simulink model "CAMFC2_04_simple_DoubleIntegrator_02"  (R2017b)
settings: Solver=ode23  StartTime=0.0  StopTime=200  RelTol=1e-3  EnableMultiTasking=on
InitFcn:
  | constant_CAMFC2_04_Simple_DoubleIntegrator_02
values from neighbouring files (symbols this model uses):
  alpha = 0.1    [constant_CAMFC2_01_WMR01.m]    (also in constant_CAMFC2_04_Comp.m = 0.01; constant_CAMFC2_04_Quad_03.m; constant_CAMFC2_04_Simple.m = 0.01; constant_CAMFC2_04_Simple_DoubleIntegrator.m = 0.01)
  AN = [     0 1 0 0 ... (first row only)    [constant_CAMFC2_01_WMR01.m]    (also in constant_CAMFC2_04_Comp.m = [     0 1 0 0 1; constant_CAMFC2_04_Quad_03.m; constant_CAMFC2_04_Simple.m; constant_CAMFC2_04_Simple_DoubleIntegrator.m)
  BN = [     1 0 0 0 ... (first row only)    [constant_CAMFC2_01_WMR01.m]    (also in constant_CAMFC2_04_Comp.m = [     0 0 0 0 0; constant_CAMFC2_04_Quad_03.m; constant_CAMFC2_04_Simple.m; constant_CAMFC2_04_Simple_DoubleIntegrator.m)
  Bp = 0.01    [constant_CAMFC2_04_Comp.m]    (also in constant_CAMFC2_04_Simple.m; constant_CAMFC2_04_Simple_DoubleIntegrator.m; constant_CAMFC2_04_Simple_DoubleIntegrator_02.m; constants_CAMFC2_Pendulum_Comp_Lewis.m)
  chi = [0 0 0 0 ... (first row only)    [constant_CAMFC2_01_WMR01.m]    (also in constant_CAMFC2_04_Comp.m = X_m*ones(n0,1); constant_CAMFC2_04_Quad_03.m = X_m*ones(n0,1); constant_CAMFC2_04_Simple.m = X_m*ones(n0,1); constant_CAMFC2_04_Simple_DoubleIntegrator.m = X_m*ones(n0,1))
  Disturb_Freq = 2    [constant_CAMFC2_04_Comp.m]    (also in constant_CAMFC2_04_Simple.m; constant_CAMFC2_04_Simple_DoubleIntegrator.m; constant_CAMFC2_04_Simple_DoubleIntegrator_02.m; constants_CAMFC2_Pendulum_Comp_Lewis.m)
  Disturb_Val = 1    [constant_CAMFC2_04_Comp.m]    (also in constant_CAMFC2_04_Simple.m; constant_CAMFC2_04_Simple_DoubleIntegrator.m; constant_CAMFC2_04_Simple_DoubleIntegrator_02.m; constants_CAMFC2_Pendulum_Comp_Lewis.m)
  epsilon_struct = struct('data',epsilon_InitVal)    [constant_CAMFC2_01_WMR01.m]    (also in constant_CAMFC2_04_Comp.m; constant_CAMFC2_04_Quad_03.m; constant_CAMFC2_04_Simple.m; constant_CAMFC2_04_Simple_DoubleIntegrator.m)
  gama1_Int1 = 1e+2*1e0    (= 100)    [constant_CAMFC2_04_Simple_DoubleIntegrator.m]    (also in constant_CAMFC2_04_Simple_DoubleIntegrator_02.m)
  gama1_Int2 = 1e+3*1e0    (= 1000)    [constant_CAMFC2_04_Simple_DoubleIntegrator.m]    (also in constant_CAMFC2_04_Simple_DoubleIntegrator_02.m)
  gama2_Int1 = 1e+0*1e0    (= 1)    [constant_CAMFC2_04_Simple_DoubleIntegrator.m]    (also in constant_CAMFC2_04_Simple_DoubleIntegrator_02.m)
  gama2_Int2 = 1e+2*1e0    (= 100)    [constant_CAMFC2_04_Simple_DoubleIntegrator.m]    (also in constant_CAMFC2_04_Simple_DoubleIntegrator_02.m)
  ge = 9.81    [constant_CAMFC2_04_Comp.m]    (also in constant_CAMFC2_04_Quad_03.m; constant_CAMFC2_04_Simple.m; constant_CAMFC2_04_Simple_DoubleIntegrator.m; constant_CAMFC2_04_Simple_DoubleIntegrator_02.m)
  H = L + BN    [constant_CAMFC2_01_WMR01.m]    (also in constant_CAMFC2_04_Comp.m; constant_CAMFC2_04_Quad_03.m; constant_CAMFC2_04_Simple.m; constant_CAMFC2_04_Simple_DoubleIntegrator.m)
  Jp = 1    [constant_CAMFC2_04_Comp.m]    (also in constant_CAMFC2_04_Simple.m; constant_CAMFC2_04_Simple_DoubleIntegrator.m; constant_CAMFC2_04_Simple_DoubleIntegrator_02.m; constants_CAMFC2_Pendulum_Comp_Lewis.m)
  k1 = 1    [constant_CAMFC2_01_WMR01.m]    (also in constant_CAMFC2_04_Comp.m; constant_CAMFC2_04_Quad_03.m = 50; constant_CAMFC2_04_Simple.m; constant_CAMFC2_04_Simple_DoubleIntegrator.m)
  k2 = 1    [constant_CAMFC2_01_WMR01.m]    (also in constant_CAMFC2_04_Comp.m; constant_CAMFC2_04_Quad_03.m; constant_CAMFC2_04_Simple.m; constant_CAMFC2_04_Simple_DoubleIntegrator.m)
  lp = 0.1    [constant_CAMFC2_04_Comp.m]    (also in constant_CAMFC2_04_Simple.m; constant_CAMFC2_04_Simple_DoubleIntegrator.m; constant_CAMFC2_04_Simple_DoubleIntegrator_02.m; constants_CAMFC2_Pendulum_Comp_Lewis.m)
  Mp = 0.1    [constant_CAMFC2_04_Comp.m]    (also in constant_CAMFC2_04_Simple.m; constant_CAMFC2_04_Simple_DoubleIntegrator.m; constant_CAMFC2_04_Simple_DoubleIntegrator_02.m; constants_CAMFC2_Pendulum_Comp_Lewis.m)
  n = 4    [constant_CAMFC2_01_WMR01.m]    (also in constant_CAMFC2_04_Comp.m = 2; constant_CAMFC2_04_Quad_03.m = 6; constant_CAMFC2_04_Simple.m = 2; constant_CAMFC2_04_Simple_DoubleIntegrator.m = 2)
  N = 4    [constant_CAMFC2_01_WMR01.m]    (also in constant_CAMFC2_04_Comp.m = 5; constant_CAMFC2_04_Quad_03.m; constant_CAMFC2_04_Simple.m; constant_CAMFC2_04_Simple_DoubleIntegrator.m)
  n0 = 2    [constant_CAMFC2_01_WMR01.m]    (also in constant_CAMFC2_04_Comp.m = 1; constant_CAMFC2_04_Quad_03.m = 3; constant_CAMFC2_04_Simple.m; constant_CAMFC2_04_Simple_DoubleIntegrator.m = 1)
  Observer_Gain = 100    [constant_CAMFC2_01_WMR01.m]    (also in constant_CAMFC2_04_Comp.m = 10; constant_CAMFC2_04_Quad_03.m = 1; constant_CAMFC2_04_Simple.m; constant_CAMFC2_04_Simple_DoubleIntegrator.m)
  Observer_Gain1 = 100    [constant_CAMFC2_01_WMR01.m]    (also in constant_CAMFC2_04_Comp.m = 10; constant_CAMFC2_04_Quad_03.m = 1; constant_CAMFC2_04_Simple.m; constant_CAMFC2_04_Simple_DoubleIntegrator.m)
  Omega = [0 0 ... (first row only)    [constant_CAMFC2_04_Comp.m]    (also in constant_CAMFC2_04_Simple.m; constant_CAMFC2_04_Simple_DoubleIntegrator.m; constant_CAMFC2_04_Simple_DoubleIntegrator_02.m; constant_CAMFC2_04_Simple_Formation.m)
  P_struct = struct('data',P_InitVal)    [constant_CAMFC2_01_WMR01.m]    (also in constant_CAMFC2_04_Comp.m; constant_CAMFC2_04_Quad_03.m; constant_CAMFC2_04_Simple.m; constant_CAMFC2_04_Simple_DoubleIntegrator.m)
  Q_Int2 = 1.0e+1    (= 10)    [constant_CAMFC2_04_Simple_DoubleIntegrator.m]    (also in constant_CAMFC2_04_Simple_DoubleIntegrator_02.m = 2)
  rho1 = 1e-1    (= 0.1)    [constant_CAMFC2_01_WMR01.m]    (also in constant_CAMFC2_04_Comp.m = 1; constant_CAMFC2_04_Quad_03.m = 1; constant_CAMFC2_04_Simple.m = 1; constant_CAMFC2_04_Simple_DoubleIntegrator.m = 1)
  rho2 = 1e-3    (= 0.001)    [constant_CAMFC2_01_WMR01.m]    (also in constant_CAMFC2_04_Comp.m = 1; constant_CAMFC2_04_Quad_03.m = 1; constant_CAMFC2_04_Simple.m = 1; constant_CAMFC2_04_Simple_DoubleIntegrator.m = 10)
  T_struct = struct('data',T_InitVal)    [constant_CAMFC2_01_WMR01.m]    (also in constant_CAMFC2_04_Comp.m; constant_CAMFC2_04_Quad_03.m; constant_CAMFC2_04_Simple.m; constant_CAMFC2_04_Simple_DoubleIntegrator.m)
  Upsilon_M = Upsilon_m*ones(n,1)    [constant_CAMFC2_01_WMR01.m]    (also in constant_CAMFC2_04_Comp.m; constant_CAMFC2_04_Quad_03.m = Upsilon_m*ones(n0,1); constant_CAMFC2_04_Simple.m; constant_CAMFC2_04_Simple_DoubleIntegrator.m)
(part 1 of 4)
settings Model: ExtModeTrigDuration=100  Creator=hp  LastModifiedBy=ali.safaei
settings DataIOCC: LimitDataPoints=on  SaveFinalState=on  SaveFormat=StructureWithTime  SaveOutput=off  SaveState=on  StateSaveName=tmp_raccel_xout  SignalLoggingName=tmp_raccel_logsout
settings OptimizationCC: EfficientMapNaN2IntZero=off  LifeSpan=inf
settings DebuggingCC: UnderspecifiedInitializationDetection=Classic  MergeDetectMultiDrivingBlocksExec=none  SFUnexpectedBacktrackingDiag=warning  SFNoUnconditionalDefaultTransitionDiag=warning  SFExecutionAtInitializationDiag=none
settings HardwareCC: ProdBitPerPointer=32  ProdBitPerSizeT=32  ProdBitPerPtrDiffT=32  ProdLargestAtomicFloat=None  ProdIntDivRoundTo=Undefined  ProdEndianess=Unspecified  ProdWordSize=32  ProdHWDeviceType=32-bit Generic  TargetBitPerPointer=64  TargetBitPerSizeT=64  TargetBitPerPtrDiffT=64  TargetLongLongMode=on  TargetIntDivRoundTo=Zero  TargetEndianess=LittleEndian  TargetWordSize=64  TargetHWDeviceType=MATLAB Host  ProdEqTarget=off
settings ModelReferenceCC: PropagateSignalLabelsOutOfModel=off
settings RTWCC: SystemTargetFile=raccel.tlc  TemplateMakefile=raccel_default_tmf  RTWVerbose=off  RTWUseSimCustomCode=on
settings CodeAppCC: GenerateComments=off  MaxIdLength=128  MangleLength=10  SimulinkBlockComments=off
settings RaccelTargetCC: GeneratePreprocessorConditionals=Use local settings  MultiInstanceERTCode=off  ExtModeMexArgs='', 0, 54523  ENABLE_SLEXEC_SSBRIDGE=0  RTWCAPIParams=on
settings ConfigComp: CovMetricSettings=dw  CovHtmlReporting=on  CovSaveCumulativeToWorkspaceVar=on  CovSaveSingleToWorkspaceVar=on  CovExternalEMLEnable=off

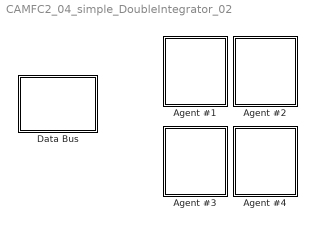
== system CAMFC2_04_simple_DoubleIntegrator_02 ==
  Agent #1 : Subsystem
  Agent #2 : Subsystem
  Agent #3 : Subsystem
  Agent #4 : Subsystem
  "Data Bus " : Subsystem

== system CAMFC2_04_simple_DoubleIntegrator_02/Agent #1 ==
  Agent # : Constant
  Controller interpreter #1 : MATLAB Function  TreatAsAtomicUnit=on
  Decenteralized Cooperaive Controller #1 : Subsystem
  Pendulum Plant #1 : Subsystem
  tag scope: u1=global, x1=global
  wires:
  Decenteralized Cooperaive Controller #1/1(U1) -> Controller interpreter #1/1(U)
  Agent #/1 -> Decenteralized Cooperaive Controller #1/1(Agent_Num)
  Pendulum Plant #1/1(Y) -> [x1]
  Controller interpreter #1/1(u) -> [u1], Pendulum Plant #1/1(U)

== system CAMFC2_04_simple_DoubleIntegrator_02/Agent #2 ==
  Agent # : Constant  Value=2
  Controller interpreter #2 : MATLAB Function  TreatAsAtomicUnit=on
  Decenteralized Cooperaive Controller #2 : Subsystem
  Pendulum Plant #2 : Subsystem
  tag scope: u2=global, x2=global
  wires:
  Controller interpreter #2/1(u) -> Pendulum Plant #2/1(U), [u2]
  Pendulum Plant #2/1(Y) -> [x2]
  Agent #/1 -> Decenteralized Cooperaive Controller #2/1(Agent_Num)
  Decenteralized Cooperaive Controller #2/1(U2) -> Controller interpreter #2/1(U)

== system CAMFC2_04_simple_DoubleIntegrator_02/Agent #3 ==
  Agent # : Constant  Value=3
  Controller interpreter #3 : MATLAB Function  TreatAsAtomicUnit=on
  Decenteralized Cooperaive Controller #3 : Subsystem
  Pendulum Plant #3 : Subsystem
  tag scope: u3=global, x3=global
  wires:
  Decenteralized Cooperaive Controller #3/1(U3) -> Controller interpreter #3/1(U)
  Agent #/1 -> Decenteralized Cooperaive Controller #3/1(Agent_Num)
  Pendulum Plant #3/1(Y) -> [x3]
  Controller interpreter #3/1(u) -> [u3], Pendulum Plant #3/1(U)

== system CAMFC2_04_simple_DoubleIntegrator_02/Agent #4 ==
  Agent # : Constant  Value=4
  Controller interpreter #4 : MATLAB Function  TreatAsAtomicUnit=on
  Decenteralized Cooperaive Controller #4 : Subsystem
  Pendulum Plant #4 : Subsystem
  tag scope: u4=global, x4=global
  wires:
  Controller interpreter #4/1(u) -> Pendulum Plant #4/1(U), [u4]
  Pendulum Plant #4/1(Y) -> [x4]
  Agent #/1 -> Decenteralized Cooperaive Controller #4/1(Agent_Num)
  Decenteralized Cooperaive Controller #4/1(U4) -> Controller interpreter #4/1(U)

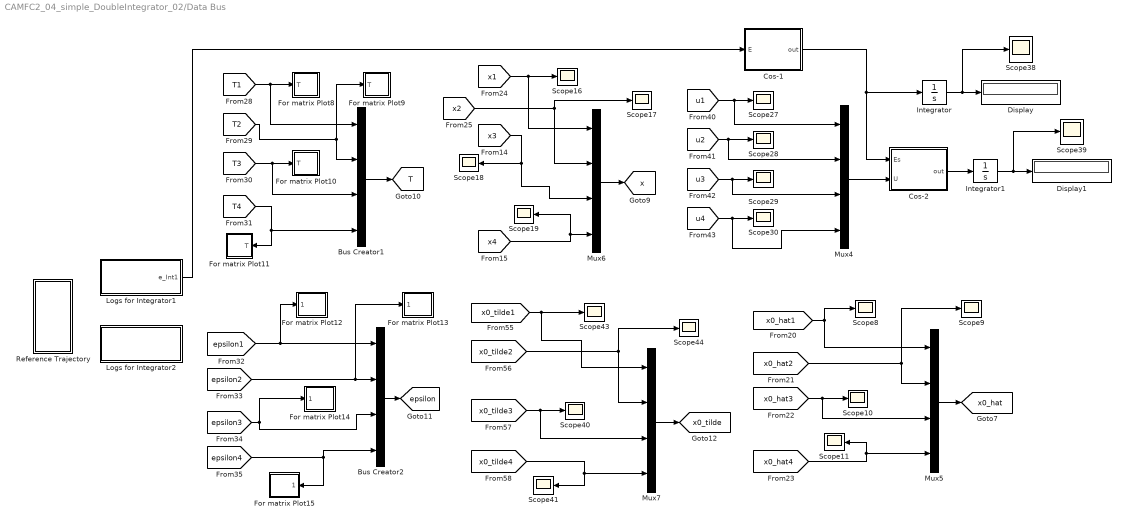
== system CAMFC2_04_simple_DoubleIntegrator_02/Data Bus  ==
  Bus Creator1 : BusCreator  Inputs=4  OutDataTypeStr=Bus: T_bus
  Bus Creator2 : BusCreator  Inputs=4  OutDataTypeStr=Bus: epsilon_bus
  Cos-1 : MATLAB Function  TreatAsAtomicUnit=on
  Cos-2 : MATLAB Function  TreatAsAtomicUnit=on
  Display : Display
  Display1 : Display
  For matrix Plot10 : Subsystem
  For matrix Plot11 : Subsystem
  For matrix Plot12 : Subsystem
  For matrix Plot13 : Subsystem
  For matrix Plot14 : Subsystem
  For matrix Plot15 : Subsystem
  For matrix Plot8 : Subsystem
  For matrix Plot9 : Subsystem
  Integrator : Integrator
  Integrator1 : Integrator
  Logs for Integrator1 : Subsystem
  Logs for Integrator2 : Subsystem
  Mux{4..7} (4 alike) : Mux
  Reference Trajectory : Subsystem
  Scope{8..11,16..19,27..30,38..41,43..44} (18 alike) : Scope
  tag scope: T=global, epsilon=global, x0_hat=global, x0_tilde=global, x=global
  wires:
  [x0_hat2] -> Scope9/1, Mux5/2
  [x0_hat1] -> Scope8/1, Mux5/1
  Mux5/1 -> [x0_hat]
  [x2] -> Scope17/1, Mux6/2
  [x1] -> Mux6/1, Scope16/1
  Mux6/1 -> [x]
  [x3] -> Scope18/1, Mux6/3
  [x4] -> Scope19/1, Mux6/4
  [x0_hat3] -> Mux5/3, Scope10/1
  [x0_hat4] -> Mux5/4, Scope11/1
  [T2] -> For matrix Plot9/1(T), Bus Creator1/2
  [T1] -> Bus Creator1/1, For matrix Plot8/1(T)
  Bus Creator1/1 -> [T]
  [T3] -> Bus Creator1/3, For matrix Plot10/1(T)
  [T4] -> Bus Creator1/4, For matrix Plot11/1(T)
  [epsilon2] -> For matrix Plot13/1(epsilon), Bus Creator2/2
  [epsilon1] -> For matrix Plot12/1(epsilon), Bus Creator2/1
  Bus Creator2/1 -> [epsilon]
  [epsilon3] -> For matrix Plot14/1(epsilon), Bus Creator2/3
  [epsilon4] -> Bus Creator2/4, For matrix Plot15/1(epsilon)
  [u2] -> Mux4/2, Scope28/1
  [u1] -> Mux4/1, Scope27/1
  [u4] -> Mux4/4, Scope30/1
  [u3] -> Mux4/3, Scope29/1
  [x0_tilde4] -> Mux7/4, Scope41/1
  [x0_tilde1] -> Mux7/1, Scope43/1
  [x0_tilde3] -> Mux7/3, Scope40/1
  [x0_tilde2] -> Mux7/2, Scope44/1
  Mux7/1 -> [x0_tilde]
  Cos-2/1(out) -> Integrator1/1
  Integrator1/1 -> Display1/1, Scope39/1
  Logs for Integrator1/1(e_Int1) -> Cos-1/1(E)
  Cos-1/1(out) -> Cos-2/1(Es), Integrator/1
  Mux4/1 -> Cos-2/2(U)
  Integrator/1 -> Scope38/1, Display/1

== system CAMFC2_04_simple_DoubleIntegrator_02/Agent #1/Decenteralized Cooperaive Controller #1 ==
  Agent_Num : Inport
  Cooperative observer for formation variables #1 : Subsystem
  Cooperative observer for leader states #1 : Subsystem
  Differentiator1 : Subsystem
  First Integrator #1 : Subsystem
  Second Integrator #1 : Subsystem
  formation topology for second integrator : MATLAB Function  TreatAsAtomicUnit=on
  U1 : Outport
  tag scope: U1_Int1=global
  wires:
  Agent_Num/1 -> Cooperative observer for leader states #1/1(Agent_Num), Cooperative observer for formation variables #1/1(Agent_Num), First Integrator #1/1(Agent Num), Second Integrator #1/1(Agent_Num)
  Second Integrator #1/1(U) -> U1/1
  Cooperative observer for leader states #1/1(x0_hat_i) -> Differentiator1/1(x_d), First Integrator #1/2(x0_hat_i)
  Cooperative observer for formation variables #1/1(T_i) -> formation topology for second integrator/1(T_i), First Integrator #1/3(T_i)
  First Integrator #1/1(U to Second Integrator) -> [U1_Int1]
  [U_Int1] -> formation topology for second integrator/2(U_Int1)
  formation topology for second integrator/1(New_T_i) -> Second Integrator #1/3(T_i)
  Differentiator1/1(Dx_d) -> Second Integrator #1/2(Dx0_hat_i)

== system CAMFC2_04_simple_DoubleIntegrator_02/Agent #1/Pendulum Plant #1 ==
  U : Inport
  Plant : Subsystem
  Y : Outport
  wires:
  U/1 -> Plant/1(U)
  Plant/1(Y) -> Y/1

== system CAMFC2_04_simple_DoubleIntegrator_02/Agent #2/Decenteralized Cooperaive Controller #2 ==
  Agent_Num : Inport
  Cooperative observer for formation variables #2 : Subsystem
  Cooperative observer for leader states #2 : Subsystem
  Differentiator1 : Subsystem
  First Integrator #2 : Subsystem
  Second Integrator #2 : Subsystem
  formation topology for second integrator : MATLAB Function  TreatAsAtomicUnit=on
  U2 : Outport
  tag scope: U2_Int1=global
  wires:
  Cooperative observer for leader states #2/1(x0_hat_i) -> Differentiator1/1(x_d), First Integrator #2/2(x0_hat_i)
  Second Integrator #2/1(U) -> U2/1
  Agent_Num/1 -> Cooperative observer for formation variables #2/1(Agent_Num), Cooperative observer for leader states #2/1(Agent_Num), First Integrator #2/1(Agent Num), Second Integrator #2/1(Agent_Num)
  First Integrator #2/1(U to Second Integrator) -> [U2_Int1]
  formation topology for second integrator/1(New_T_i) -> Second Integrator #2/3(T_i)
  Cooperative observer for formation variables #2/1(T_i) -> First Integrator #2/3(T_i), formation topology for second integrator/1(T_i)
  [U_Int1] -> formation topology for second integrator/2(U_Int1)
  Differentiator1/1(Dx_d) -> Second Integrator #2/2(Dx0_hat_i)

== system CAMFC2_04_simple_DoubleIntegrator_02/Agent #2/Pendulum Plant #2 ==
  U : Inport
  Plant : Subsystem
  Y : Outport
  wires:
  Plant/1(Y) -> Y/1
  U/1 -> Plant/1(U)

== system CAMFC2_04_simple_DoubleIntegrator_02/Agent #3/Decenteralized Cooperaive Controller #3 ==
  Agent_Num : Inport
  Cooperative observer for formation variables #3 : Subsystem
  Cooperative observer for leader states #3 : Subsystem
  Differentiator1 : Subsystem
  First Integrator #3 : Subsystem
  Second Integrator #3 : Subsystem
  formation topology for second integrator : MATLAB Function  TreatAsAtomicUnit=on
  U3 : Outport
  tag scope: U3_Int1=global
  wires:
  Agent_Num/1 -> Cooperative observer for leader states #3/1(Agent_Num), Cooperative observer for formation variables #3/1(Agent_Num), First Integrator #3/1(Agent Num), Second Integrator #3/1(Agent_Num)
  Second Integrator #3/1(U) -> U3/1
  Cooperative observer for leader states #3/1(x0_hat_i) -> Differentiator1/1(x_d), First Integrator #3/2(x0_hat_i)
  First Integrator #3/1(U to Second Integrator) -> [U3_Int1]
  formation topology for second integrator/1(New_T_i) -> Second Integrator #3/3(T_i)
  Cooperative observer for formation variables #3/1(T_i) -> First Integrator #3/3(T_i), formation topology for second integrator/1(T_i)
  [U_Int1] -> formation topology for second integrator/2(U_Int1)
  Differentiator1/1(Dx_d) -> Second Integrator #3/2(Dx0_hat_i)

== system CAMFC2_04_simple_DoubleIntegrator_02/Agent #3/Pendulum Plant #3 ==
  U : Inport
  Plant : Subsystem
  Y : Outport
  wires:
  U/1 -> Plant/1(U)
  Plant/1(Y) -> Y/1

== system CAMFC2_04_simple_DoubleIntegrator_02/Agent #4/Decenteralized Cooperaive Controller #4 ==
  Agent_Num : Inport
  Cooperative observer for formation variables #4 : Subsystem
  Cooperative observer for leader states #4 : Subsystem
  Differentiator1 : Subsystem
  First Integrator #4 : Subsystem
  Second Integrator #4 : Subsystem
  formation topology for second integrator : MATLAB Function  TreatAsAtomicUnit=on
  U4 : Outport
  tag scope: U4_Int1=global
  wires:
  Cooperative observer for leader states #4/1(x0_hat_i) -> Differentiator1/1(x_d), First Integrator #4/2(x0_hat_i)
  Second Integrator #4/1(U) -> U4/1
  Agent_Num/1 -> First Integrator #4/1(Agent Num), Cooperative observer for formation variables #4/1(Agent_Num), Cooperative observer for leader states #4/1(Agent_Num), Second Integrator #4/1(Agent_Num)
  First Integrator #4/1(U to Second Integrator) -> [U4_Int1]
  formation topology for second integrator/1(New_T_i) -> Second Integrator #4/3(T_i)
  Cooperative observer for formation variables #4/1(T_i) -> First Integrator #4/3(T_i), formation topology for second integrator/1(T_i)
  [U_Int1] -> formation topology for second integrator/2(U_Int1)
  Differentiator1/1(Dx_d) -> Second Integrator #4/2(Dx0_hat_i)

== system CAMFC2_04_simple_DoubleIntegrator_02/Agent #4/Pendulum Plant #4 ==
  U : Inport
  Plant : Subsystem
  Y : Outport
  wires:
  Plant/1(Y) -> Y/1
  U/1 -> Plant/1(U)

== system CAMFC2_04_simple_DoubleIntegrator_02/Data Bus /For matrix Plot10 ==
  T : Inport
  MATLAB Function : MATLAB Function  TreatAsAtomicUnit=on
  To Workspace : ToWorkspace  VariableName=T3  SaveFormat=Structure With Time  SampleTime=-1
  wires:
  T/1 -> MATLAB Function/1(u)
  MATLAB Function/1(y) -> To Workspace/1

== system CAMFC2_04_simple_DoubleIntegrator_02/Data Bus /For matrix Plot11 ==
  T : Inport
  MATLAB Function : MATLAB Function  TreatAsAtomicUnit=on
  To Workspace : ToWorkspace  VariableName=T4  SaveFormat=Structure With Time  SampleTime=-1
  wires:
  MATLAB Function/1(y) -> To Workspace/1
  T/1 -> MATLAB Function/1(u)

== system CAMFC2_04_simple_DoubleIntegrator_02/Data Bus /For matrix Plot12 ==
  epsilon : Inport
  MATLAB Function : MATLAB Function  TreatAsAtomicUnit=on
  To Workspace : ToWorkspace  VariableName=epsilon1  SaveFormat=Structure With Time  SampleTime=-1
  wires:
  epsilon/1 -> MATLAB Function/1(u)
  MATLAB Function/1(y) -> To Workspace/1

== system CAMFC2_04_simple_DoubleIntegrator_02/Data Bus /For matrix Plot13 ==
  epsilon : Inport
  MATLAB Function : MATLAB Function  TreatAsAtomicUnit=on
  To Workspace : ToWorkspace  VariableName=epsilon2  SaveFormat=Structure With Time  SampleTime=-1
  wires:
  MATLAB Function/1(y) -> To Workspace/1
  epsilon/1 -> MATLAB Function/1(u)

== system CAMFC2_04_simple_DoubleIntegrator_02/Data Bus /For matrix Plot14 ==
  epsilon : Inport
  MATLAB Function : MATLAB Function  TreatAsAtomicUnit=on
  To Workspace : ToWorkspace  VariableName=epsilon3  SaveFormat=Structure With Time  SampleTime=-1
  wires:
  MATLAB Function/1(y) -> To Workspace/1
  epsilon/1 -> MATLAB Function/1(u)

== system CAMFC2_04_simple_DoubleIntegrator_02/Data Bus /For matrix Plot15 ==
  epsilon : Inport
  MATLAB Function : MATLAB Function  TreatAsAtomicUnit=on
  To Workspace : ToWorkspace  VariableName=epsilon4  SaveFormat=Structure With Time  SampleTime=-1
  wires:
  epsilon/1 -> MATLAB Function/1(u)
  MATLAB Function/1(y) -> To Workspace/1

== system CAMFC2_04_simple_DoubleIntegrator_02/Data Bus /For matrix Plot8 ==
  T : Inport
  MATLAB Function : MATLAB Function  TreatAsAtomicUnit=on
  Scope17 : Scope
  To Workspace : ToWorkspace  VariableName=T1  SaveFormat=Structure With Time  SampleTime=-1
  wires:
  MATLAB Function/1(y) -> Scope17/1, To Workspace/1
  T/1 -> MATLAB Function/1(u)

== system CAMFC2_04_simple_DoubleIntegrator_02/Data Bus /For matrix Plot9 ==
  T : Inport
  MATLAB Function : MATLAB Function  TreatAsAtomicUnit=on
  To Workspace : ToWorkspace  VariableName=T2  SaveFormat=Structure With Time  SampleTime=-1
  wires:
  T/1 -> MATLAB Function/1(u)
  MATLAB Function/1(y) -> To Workspace/1

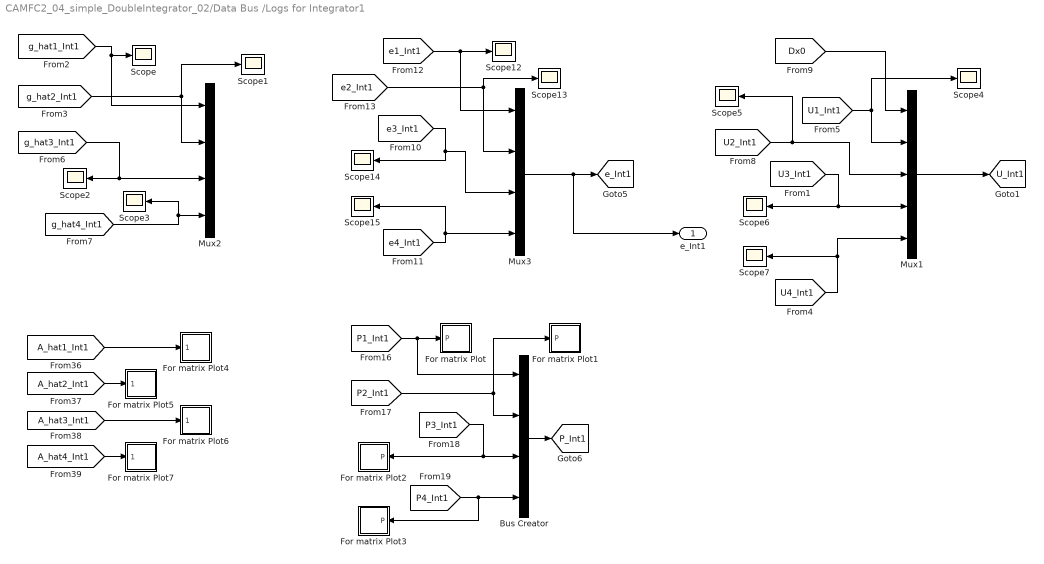
== system CAMFC2_04_simple_DoubleIntegrator_02/Data Bus /Logs for Integrator1 ==
  Bus Creator : BusCreator  Inputs=4  OutDataTypeStr=Bus: P_bus
  For matrix Plot : Subsystem
  For matrix Plot1 : Subsystem
  For matrix Plot2 : Subsystem
  For matrix Plot3 : Subsystem
  For matrix Plot4 : Subsystem
  For matrix Plot5 : Subsystem
  For matrix Plot6 : Subsystem
  For matrix Plot7 : Subsystem
  Mux1 : Mux  Inputs=5
  Mux2 : Mux
  Mux3 : Mux
  Scope{,1..7,12..15} (12 alike) : Scope
  e_Int1 : Outport
  tag scope: P_Int1=global, U_Int1=global, e_Int1=global
  wires:
  [g_hat1_Int1] -> Mux2/1, Scope/1
  Mux3/1 -> e_Int1/1, [e_Int1]
  [e3_Int1] -> Scope14/1, Mux3/3
  [g_hat3_Int1] -> Scope2/1, Mux2/3
  [e2_Int1] -> Scope13/1, Mux3/2
  [g_hat4_Int1] -> Scope3/1, Mux2/4
  [e1_Int1] -> Mux3/1, Scope12/1
  [g_hat2_Int1] -> Mux2/2, Scope1/1
  [e4_Int1] -> Scope15/1, Mux3/4
  [P4_Int1] -> For matrix Plot3/1(P), Bus Creator/4
  [P3_Int1] -> For matrix Plot2/1(P), Bus Creator/3
  [P1_Int1] -> Bus Creator/1, For matrix Plot/1(P)
  Bus Creator/1 -> [P_Int1]
  [P2_Int1] -> Bus Creator/2, For matrix Plot1/1(P)
  [A_hat3_Int1] -> For matrix Plot6/1(A_hat)
  [A_hat2_Int1] -> For matrix Plot5/1(A_hat)
  [A_hat4_Int1] -> For matrix Plot7/1(A_hat)
  [A_hat1_Int1] -> For matrix Plot4/1(A_hat)
  [U2_Int1] -> Mux1/3, Scope5/1
  [U1_Int1] -> Scope4/1, Mux1/2
  [U4_Int1] -> Scope7/1, Mux1/5
  [U3_Int1] -> Mux1/4, Scope6/1
  Mux1/1 -> [U_Int1]
  [Dx0] -> Mux1/1

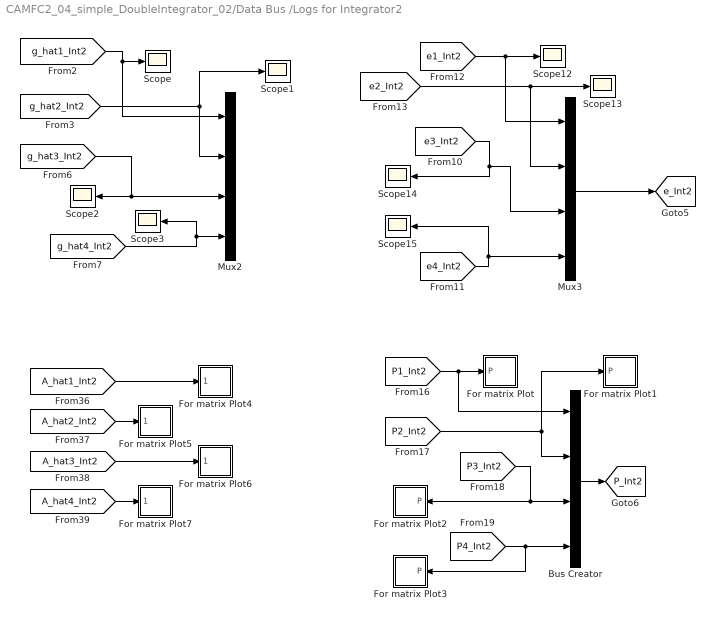
== system CAMFC2_04_simple_DoubleIntegrator_02/Data Bus /Logs for Integrator2 ==
  Bus Creator : BusCreator  Inputs=4  OutDataTypeStr=Bus: P_bus
  For matrix Plot : Subsystem
  For matrix Plot1 : Subsystem
  For matrix Plot2 : Subsystem
  For matrix Plot3 : Subsystem
  For matrix Plot4 : Subsystem
  For matrix Plot5 : Subsystem
  For matrix Plot6 : Subsystem
  For matrix Plot7 : Subsystem
  Mux2 : Mux
  Mux3 : Mux
  Scope{,1..3,12..15} (8 alike) : Scope
  tag scope: P_Int2=global, e_Int2=global
  wires:
  [A_hat4_Int2] -> For matrix Plot7/1(A_hat)
  [A_hat1_Int2] -> For matrix Plot4/1(A_hat)
  Bus Creator/1 -> [P_Int2]
  [P1_Int2] -> Bus Creator/1, For matrix Plot/1(P)
  [P4_Int2] -> For matrix Plot3/1(P), Bus Creator/4
  [P2_Int2] -> Bus Creator/2, For matrix Plot1/1(P)
  [A_hat3_Int2] -> For matrix Plot6/1(A_hat)
  [e1_Int2] -> Mux3/1, Scope12/1
  [g_hat4_Int2] -> Scope3/1, Mux2/4
  [e2_Int2] -> Mux3/2, Scope13/1
  [P3_Int2] -> For matrix Plot2/1(P), Bus Creator/3
  [e3_Int2] -> Scope14/1, Mux3/3
  [g_hat2_Int2] -> Mux2/2, Scope1/1
  [g_hat1_Int2] -> Mux2/1, Scope/1
  [g_hat3_Int2] -> Scope2/1, Mux2/3
  [e4_Int2] -> Scope15/1, Mux3/4
  Mux3/1 -> [e_Int2]
  [A_hat2_Int2] -> For matrix Plot5/1(A_hat)

== system CAMFC2_04_simple_DoubleIntegrator_02/Data Bus /Reference Trajectory ==
  Constant : Constant  Value=0
  Constant1 : Constant  Value=0
  Constant2 : Constant  Value=2
  Constant3 : Constant  Value=20
  Constant4 : Constant  Value=0
  Constant5 : Constant  Value=2
  Differentiator1 : Subsystem
  Pulse Generator : DiscretePulseGenerator  PulseType=Time based  Amplitude=2  Period=60  PulseWidth=50
  Scope1 : Scope  NumInputPorts=3
  Scope2 : Scope
  Scope26 : Scope
  X1 : Sin  Amplitude=3  Frequency=0.1  SampleTime=0
  X2 : Sin  Amplitude=3  Frequency=0.5  Phase=pi/2  SampleTime=0
  tag scope: Dx0=global, x0=global
  wires:
  Constant/1 -> Scope1/1
  Constant1/1 -> Scope1/2
  X2/1 -> Differentiator1/1(x_d), Scope26/1, [x0], Scope1/3
  Differentiator1/1(Dx_d) -> Scope2/1, [Dx0]

== system CAMFC2_04_simple_DoubleIntegrator_02/Agent #1/Decenteralized Cooperaive Controller #1/Cooperative observer for formation variables #1 ==
  Agent_Num : Inport
  Integrator5 : Integrator  InitialCondition=zeros(N+1,n)
  Memory3 : Memory  InitialCondition=zeros(N+1,n)
  Observer T#1 : MATLAB Function  TreatAsAtomicUnit=on
  T_i : Outport
  tag scope: T1=global, epsilon1=global
  wires:
  Integrator5/1 -> Observer T#1/3(T_i), [T1], T_i/1
  [T] -> Observer T#1/1(T)
  Memory3/1 -> [epsilon1]
  Observer T#1/1(DT_i) -> Integrator5/1
  [epsilon] -> Observer T#1/2(epsilon)
  Observer T#1/2(epsilon_i) -> Memory3/1
  Agent_Num/1 -> Observer T#1/4(Agent_Num)

== system CAMFC2_04_simple_DoubleIntegrator_02/Agent #1/Decenteralized Cooperaive Controller #1/Cooperative observer for leader states #1 ==
  Agent_Num : Inport
  Integrator6 : Integrator  InitialCondition=zeros(n0,1)
  Memory1 : Memory  InitialCondition=zeros(n0,1)
  Observer x0_hat#1 : MATLAB Function  TreatAsAtomicUnit=on
  x0_hat_i : Outport
  tag scope: x0_hat1=global, x0_tilde1=global
  wires:
  [x0_hat] -> Observer x0_hat#1/1(x0_hat)
  [x0_tilde] -> Observer x0_hat#1/2(x0_tilde)
  Integrator6/1 -> Observer x0_hat#1/3(x0_hat_i), [x0_hat1], x0_hat_i/1
  Observer x0_hat#1/2(x0_tilde_i) -> Memory1/1
  Agent_Num/1 -> Observer x0_hat#1/5(Agent_Num)
  Memory1/1 -> [x0_tilde1]
  Observer x0_hat#1/1(Dx0_hat_i) -> Integrator6/1
  [x0] -> Observer x0_hat#1/4(x0)

== system CAMFC2_04_simple_DoubleIntegrator_02/Agent #1/Decenteralized Cooperaive Controller #1/Differentiator1 ==
  x_d : Inport
  Integrator : Integrator  InitialCondition=zeros(n0,1)
  Integrator1 : Integrator  InitialCondition=zeros(n0,1)
  Sliding differentiator : MATLAB Function  TreatAsAtomicUnit=on
  Sliding differentiator1 : MATLAB Function  TreatAsAtomicUnit=on
  Sum : Sum  Inputs=|-+
  Dx_d : Outport
  wires:
  Sliding differentiator/1(u) -> Integrator1/1, Dx_d/1
  Sliding differentiator1/1(Du1) -> Integrator/1
  Integrator/1 -> Sliding differentiator/1(u1)
  x_d/1 -> Sum/1
  Sum/1 -> Sliding differentiator/2(e), Sliding differentiator1/1(e)
  Integrator1/1 -> Sum/2

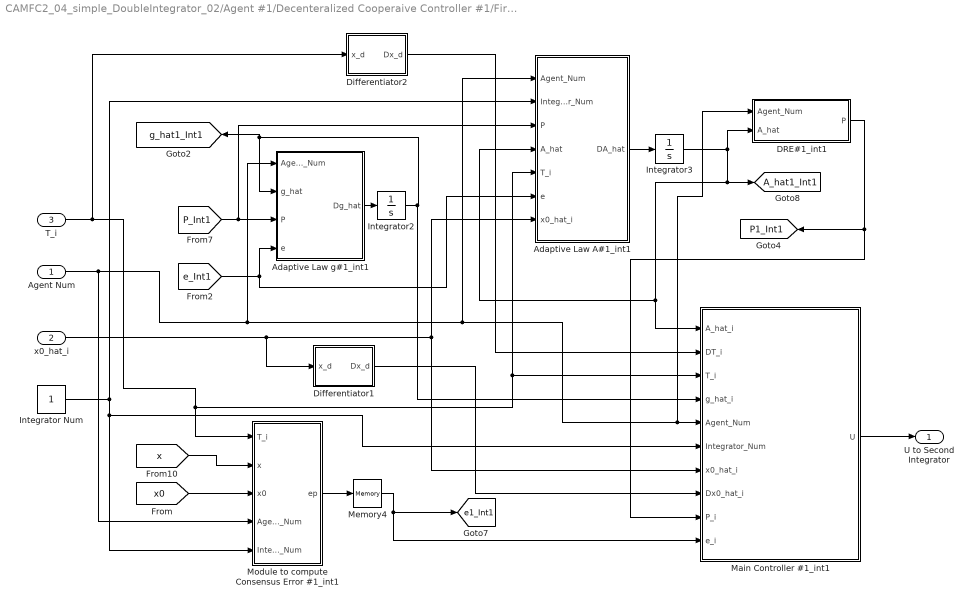
== system CAMFC2_04_simple_DoubleIntegrator_02/Agent #1/Decenteralized Cooperaive Controller #1/First Integrator #1 ==
  Agent Num : Inport
  x0_hat_i : Inport  Port=2
  T_i : Inport  Port=3
  Adaptive Law A#1_int1 : MATLAB Function  TreatAsAtomicUnit=on
  Adaptive Law g#1_int1 : MATLAB Function  TreatAsAtomicUnit=on
  DRE#1_int1 : Subsystem
  Differentiator1 : Subsystem
  Differentiator2 : Subsystem
  Integrator Num : Constant
  Integrator2 : Integrator  InitialCondition=zeros(n0,1)
  Integrator3 : Integrator  InitialCondition=zeros(n0)
  Main Controller #1_int1 : MATLAB Function  TreatAsAtomicUnit=on
  Memory4 : Memory  InitialCondition=zeros(n0,1)
  Module to compute Consensus Error #1_int1 : MATLAB Function  TreatAsAtomicUnit=on
  U to Second Integrator : Outport
  tag scope: A_hat1_Int1=global, P1_Int1=global, e1_Int1=global, g_hat1_Int1=global
  wires:
  DRE#1_int1/1(P) -> [P1_Int1], Main Controller #1_int1/9(P_i)
  Agent Num/1 -> Module to compute Consensus Error #1_int1/4(Agent_Num), Adaptive Law g#1_int1/1(Agent_Num), DRE#1_int1/1(Agent_Num), Main Controller #1_int1/5(Agent_Num), Adaptive Law A#1_int1/1(Agent_Num)
  Integrator2/1 -> Main Controller #1_int1/4(g_hat_i), Adaptive Law g#1_int1/2(g_hat), [g_hat1_Int1]
  Adaptive Law g#1_int1/1(Dg_hat) -> Integrator2/1
  Integrator3/1 -> DRE#1_int1/2(A_hat), Adaptive Law A#1_int1/4(A_hat), Main Controller #1_int1/1(A_hat_i), [A_hat1_Int1]
  Main Controller #1_int1/1(U) -> U to Second Integrator/1
  Adaptive Law A#1_int1/1(DA_hat) -> Integrator3/1
  Module to compute Consensus Error #1_int1/1(ep) -> Memory4/1
  [P_Int1] -> Adaptive Law A#1_int1/3(P), Adaptive Law g#1_int1/3(P)
  [e_Int1] -> Adaptive Law A#1_int1/6(e), Adaptive Law g#1_int1/4(e)
  [x0] -> Module to compute Consensus Error #1_int1/3(x0)
  Memory4/1 -> [e1_Int1], Main Controller #1_int1/10(e_i)
  [x] -> Module to compute Consensus Error #1_int1/2(x)
  Integrator Num/1 -> Main Controller #1_int1/6(Integrator_Num), Module to compute Consensus Error #1_int1/5(Integrator_Num), Adaptive Law A#1_int1/2(Integrator_Num)
  x0_hat_i/1 -> Differentiator1/1(x_d), Adaptive Law A#1_int1/7(x0_hat_i), Main Controller #1_int1/7(x0_hat_i)
  T_i/1 -> Differentiator2/1(x_d), Adaptive Law A#1_int1/5(T_i), Main Controller #1_int1/3(T_i), Module to compute Consensus Error #1_int1/1(T_i)
  Differentiator1/1(Dx_d) -> Main Controller #1_int1/8(Dx0_hat_i)
  Differentiator2/1(Dx_d) -> Main Controller #1_int1/2(DT_i)

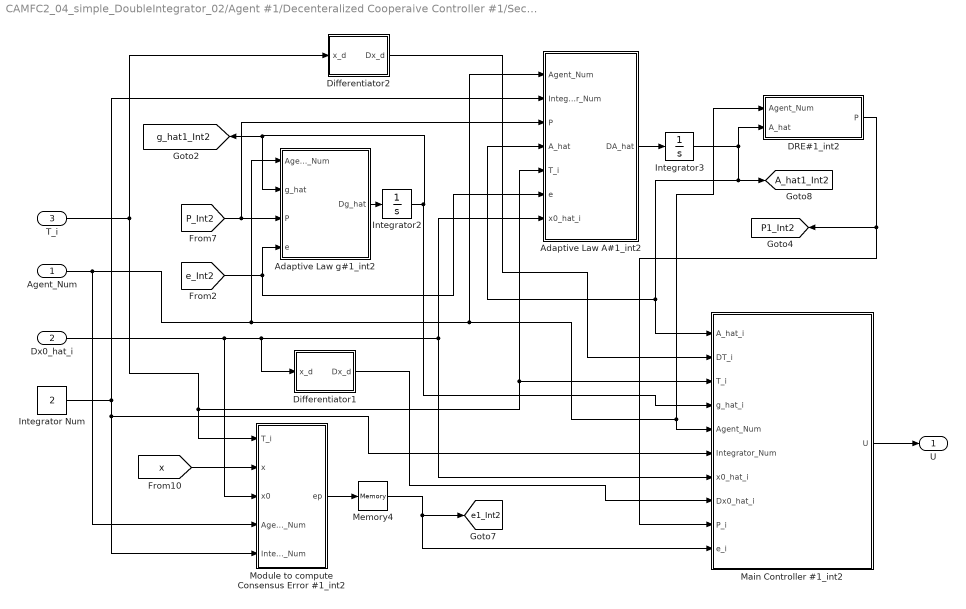
== system CAMFC2_04_simple_DoubleIntegrator_02/Agent #1/Decenteralized Cooperaive Controller #1/Second Integrator #1 ==
  Agent_Num : Inport
  Dx0_hat_i : Inport  Port=2
  T_i : Inport  Port=3
  Adaptive Law A#1_int2 : MATLAB Function  TreatAsAtomicUnit=on
  Adaptive Law g#1_int2 : MATLAB Function  TreatAsAtomicUnit=on
  DRE#1_int2 : Subsystem
  Differentiator1 : Subsystem
  Differentiator2 : Subsystem
  Integrator Num : Constant  Value=2
  Integrator2 : Integrator  InitialCondition=zeros(n0,1)
  Integrator3 : Integrator  InitialCondition=zeros(n0)
  Main Controller #1_int2 : MATLAB Function  TreatAsAtomicUnit=on
  Memory4 : Memory  InitialCondition=zeros(n0,1)
  Module to compute Consensus Error #1_int2 : MATLAB Function  TreatAsAtomicUnit=on
  U : Outport
  tag scope: A_hat1_Int2=global, P1_Int2=global, e1_Int2=global, g_hat1_Int2=global
  wires:
  [x] -> Module to compute Consensus Error #1_int2/2(x)
  Memory4/1 -> [e1_Int2], Main Controller #1_int2/10(e_i)
  Module to compute Consensus Error #1_int2/1(ep) -> Memory4/1
  [P_Int2] -> Adaptive Law A#1_int2/3(P), Adaptive Law g#1_int2/3(P)
  [e_Int2] -> Adaptive Law A#1_int2/6(e), Adaptive Law g#1_int2/4(e)
  Differentiator2/1(Dx_d) -> Main Controller #1_int2/2(DT_i)
  Adaptive Law A#1_int2/1(DA_hat) -> Integrator3/1
  Integrator3/1 -> DRE#1_int2/2(A_hat), Adaptive Law A#1_int2/4(A_hat), Main Controller #1_int2/1(A_hat_i), [A_hat1_Int2]
  Adaptive Law g#1_int2/1(Dg_hat) -> Integrator2/1
  Integrator2/1 -> Main Controller #1_int2/4(g_hat_i), Adaptive Law g#1_int2/2(g_hat), [g_hat1_Int2]
  Agent_Num/1 -> Adaptive Law g#1_int2/1(Agent_Num), DRE#1_int2/1(Agent_Num), Main Controller #1_int2/5(Agent_Num), Adaptive Law A#1_int2/1(Agent_Num), Module to compute Consensus Error #1_int2/4(Agent_Num)
  DRE#1_int2/1(P) -> [P1_Int2], Main Controller #1_int2/9(P_i)
  Differentiator1/1(Dx_d) -> Main Controller #1_int2/8(Dx0_hat_i)
  T_i/1 -> Differentiator2/1(x_d), Adaptive Law A#1_int2/5(T_i), Main Controller #1_int2/3(T_i), Module to compute Consensus Error #1_int2/1(T_i)
  Main Controller #1_int2/1(U) -> U/1
  Integrator Num/1 -> Main Controller #1_int2/6(Integrator_Num), Module to compute Consensus Error #1_int2/5(Integrator_Num), Adaptive Law A#1_int2/2(Integrator_Num)
  Dx0_hat_i/1 -> Module to compute Consensus Error #1_int2/3(x0), Adaptive Law A#1_int2/7(x0_hat_i), Main Controller #1_int2/7(x0_hat_i), Differentiator1/1(x_d)

== system CAMFC2_04_simple_DoubleIntegrator_02/Agent #1/Pendulum Plant #1/Plant ==
  U : Inport
  Clock : Clock
  Integrator : Integrator
  Integrator1 : Integrator
  Mux : Mux  Inputs=2
  Plant : MATLAB Function  TreatAsAtomicUnit=on
  Scope3 : Scope
  Y : Outport
  wires:
  Plant/1(Dx1) -> Integrator/1
  Integrator/1 -> Plant/1(x1), Mux/1
  Integrator1/1 -> Plant/2(x2), Mux/2
  U/1 -> Plant/3(u)
  Plant/2(Dx2) -> Integrator1/1
  Clock/1 -> Plant/4(t)
  Mux/1 -> Y/1, Scope3/1

== system CAMFC2_04_simple_DoubleIntegrator_02/Agent #2/Decenteralized Cooperaive Controller #2/Cooperative observer for formation variables #2 ==
  Agent_Num : Inport
  Integrator5 : Integrator  InitialCondition=zeros(N+1,n)
  Memory3 : Memory  InitialCondition=zeros(N+1,n)
  Observer T#2 : MATLAB Function  TreatAsAtomicUnit=on
  T_i : Outport
  tag scope: T2=global, epsilon2=global
  wires:
  Agent_Num/1 -> Observer T#2/4(Agent_Num)
  Observer T#2/2(epsilon_i) -> Memory3/1
  [epsilon] -> Observer T#2/2(epsilon)
  Observer T#2/1(DT_i) -> Integrator5/1
  Memory3/1 -> [epsilon2]
  [T] -> Observer T#2/1(T)
  Integrator5/1 -> [T2], Observer T#2/3(T_i), T_i/1

== system CAMFC2_04_simple_DoubleIntegrator_02/Agent #2/Decenteralized Cooperaive Controller #2/Cooperative observer for leader states #2 ==
  Agent_Num : Inport
  Integrator6 : Integrator  InitialCondition=zeros(n0,1)
  Memory1 : Memory  InitialCondition=zeros(n0,1)
  Observer x0_hat#2 : MATLAB Function  TreatAsAtomicUnit=on
  x0_hat_i : Outport
  tag scope: x0_hat2=global, x0_tilde2=global
  wires:
  [x0] -> Observer x0_hat#2/4(x0)
  Observer x0_hat#2/1(Dx0_hat_i) -> Integrator6/1
  Memory1/1 -> [x0_tilde2]
  Agent_Num/1 -> Observer x0_hat#2/5(Agent_Num)
  Observer x0_hat#2/2(x0_tilde_i) -> Memory1/1
  Integrator6/1 -> x0_hat_i/1, [x0_hat2], Observer x0_hat#2/3(x0_hat_i)
  [x0_tilde] -> Observer x0_hat#2/2(x0_tilde)
  [x0_hat] -> Observer x0_hat#2/1(x0_hat)

== system CAMFC2_04_simple_DoubleIntegrator_02/Agent #2/Decenteralized Cooperaive Controller #2/Differentiator1 ==
  x_d : Inport
  Integrator : Integrator  InitialCondition=zeros(n0,1)
  Integrator1 : Integrator  InitialCondition=zeros(n0,1)
  Sliding differentiator : MATLAB Function  TreatAsAtomicUnit=on
  Sliding differentiator1 : MATLAB Function  TreatAsAtomicUnit=on
  Sum : Sum  Inputs=|-+
  Dx_d : Outport
  wires:
  Integrator1/1 -> Sum/2
  Sum/1 -> Sliding differentiator1/1(e), Sliding differentiator/2(e)
  x_d/1 -> Sum/1
  Integrator/1 -> Sliding differentiator/1(u1)
  Sliding differentiator1/1(Du1) -> Integrator/1
  Sliding differentiator/1(u) -> Dx_d/1, Integrator1/1

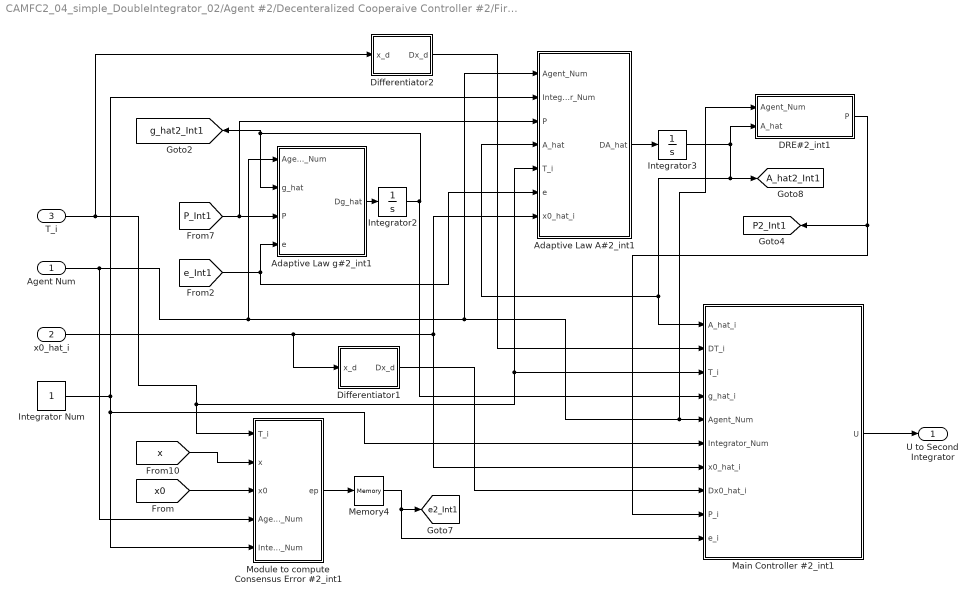
== system CAMFC2_04_simple_DoubleIntegrator_02/Agent #2/Decenteralized Cooperaive Controller #2/First Integrator #2 ==
  Agent Num : Inport
  x0_hat_i : Inport  Port=2
  T_i : Inport  Port=3
  Adaptive Law A#2_int1 : MATLAB Function  TreatAsAtomicUnit=on
  Adaptive Law g#2_int1 : MATLAB Function  TreatAsAtomicUnit=on
  DRE#2_int1 : Subsystem
  Differentiator1 : Subsystem
  Differentiator2 : Subsystem
  Integrator Num : Constant
  Integrator2 : Integrator  InitialCondition=zeros(n0,1)
  Integrator3 : Integrator  InitialCondition=zeros(n0)
  Main Controller #2_int1 : MATLAB Function  TreatAsAtomicUnit=on
  Memory4 : Memory  InitialCondition=zeros(n0,1)
  Module to compute Consensus Error #2_int1 : MATLAB Function  TreatAsAtomicUnit=on
  U to Second Integrator : Outport
  tag scope: A_hat2_Int1=global, P2_Int1=global, e2_Int1=global, g_hat2_Int1=global
  wires:
  T_i/1 -> Differentiator2/1(x_d), Module to compute Consensus Error #2_int1/1(T_i), Main Controller #2_int1/3(T_i), Adaptive Law A#2_int1/5(T_i)
  x0_hat_i/1 -> Differentiator1/1(x_d), Main Controller #2_int1/7(x0_hat_i), Adaptive Law A#2_int1/7(x0_hat_i)
  Integrator Num/1 -> Adaptive Law A#2_int1/2(Integrator_Num), Module to compute Consensus Error #2_int1/5(Integrator_Num), Main Controller #2_int1/6(Integrator_Num)
  [x] -> Module to compute Consensus Error #2_int1/2(x)
  Memory4/1 -> Main Controller #2_int1/10(e_i), [e2_Int1]
  [x0] -> Module to compute Consensus Error #2_int1/3(x0)
  [e_Int1] -> Adaptive Law g#2_int1/4(e), Adaptive Law A#2_int1/6(e)
  [P_Int1] -> Adaptive Law g#2_int1/3(P), Adaptive Law A#2_int1/3(P)
  Module to compute Consensus Error #2_int1/1(ep) -> Memory4/1
  Adaptive Law A#2_int1/1(DA_hat) -> Integrator3/1
  Main Controller #2_int1/1(U) -> U to Second Integrator/1
  Integrator3/1 -> [A_hat2_Int1], Main Controller #2_int1/1(A_hat_i), Adaptive Law A#2_int1/4(A_hat), DRE#2_int1/2(A_hat)
  Adaptive Law g#2_int1/1(Dg_hat) -> Integrator2/1
  Integrator2/1 -> [g_hat2_Int1], Adaptive Law g#2_int1/2(g_hat), Main Controller #2_int1/4(g_hat_i)
  Agent Num/1 -> Adaptive Law A#2_int1/1(Agent_Num), Main Controller #2_int1/5(Agent_Num), DRE#2_int1/1(Agent_Num), Adaptive Law g#2_int1/1(Agent_Num), Module to compute Consensus Error #2_int1/4(Agent_Num)
  DRE#2_int1/1(P) -> Main Controller #2_int1/9(P_i), [P2_Int1]
  Differentiator1/1(Dx_d) -> Main Controller #2_int1/8(Dx0_hat_i)
  Differentiator2/1(Dx_d) -> Main Controller #2_int1/2(DT_i)

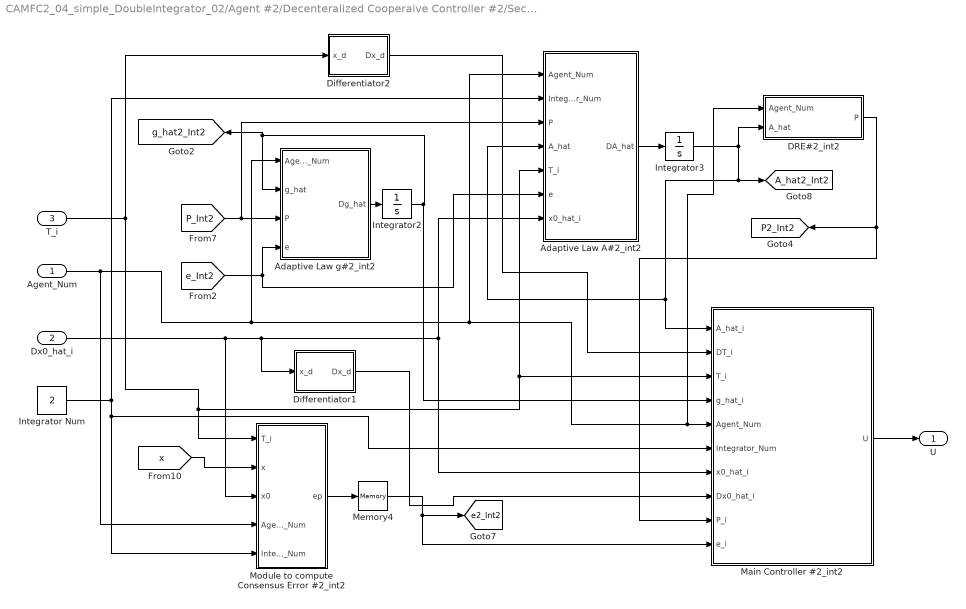
== system CAMFC2_04_simple_DoubleIntegrator_02/Agent #2/Decenteralized Cooperaive Controller #2/Second Integrator #2 ==
  Agent_Num : Inport
  Dx0_hat_i : Inport  Port=2
  T_i : Inport  Port=3
  Adaptive Law A#2_int2 : MATLAB Function  TreatAsAtomicUnit=on
  Adaptive Law g#2_int2 : MATLAB Function  TreatAsAtomicUnit=on
  DRE#2_int2 : Subsystem
  Differentiator1 : Subsystem
  Differentiator2 : Subsystem
  Integrator Num : Constant  Value=2
  Integrator2 : Integrator  InitialCondition=zeros(n0,1)
  Integrator3 : Integrator  InitialCondition=zeros(n0)
  Main Controller #2_int2 : MATLAB Function  TreatAsAtomicUnit=on
  Memory4 : Memory  InitialCondition=zeros(n0,1)
  Module to compute Consensus Error #2_int2 : MATLAB Function  TreatAsAtomicUnit=on
  U : Outport
  tag scope: A_hat2_Int2=global, P2_Int2=global, e2_Int2=global, g_hat2_Int2=global
  wires:
  Integrator Num/1 -> Adaptive Law A#2_int2/2(Integrator_Num), Module to compute Consensus Error #2_int2/5(Integrator_Num), Main Controller #2_int2/6(Integrator_Num)
  Main Controller #2_int2/1(U) -> U/1
  T_i/1 -> Module to compute Consensus Error #2_int2/1(T_i), Main Controller #2_int2/3(T_i), Adaptive Law A#2_int2/5(T_i), Differentiator2/1(x_d)
  Differentiator1/1(Dx_d) -> Main Controller #2_int2/8(Dx0_hat_i)
  DRE#2_int2/1(P) -> Main Controller #2_int2/9(P_i), [P2_Int2]
  Agent_Num/1 -> Adaptive Law A#2_int2/1(Agent_Num), Main Controller #2_int2/5(Agent_Num), DRE#2_int2/1(Agent_Num), Adaptive Law g#2_int2/1(Agent_Num), Module to compute Consensus Error #2_int2/4(Agent_Num)
  Integrator2/1 -> [g_hat2_Int2], Adaptive Law g#2_int2/2(g_hat), Main Controller #2_int2/4(g_hat_i)
  Adaptive Law g#2_int2/1(Dg_hat) -> Integrator2/1
  Integrator3/1 -> [A_hat2_Int2], Main Controller #2_int2/1(A_hat_i), Adaptive Law A#2_int2/4(A_hat), DRE#2_int2/2(A_hat)
  Adaptive Law A#2_int2/1(DA_hat) -> Integrator3/1
  Differentiator2/1(Dx_d) -> Main Controller #2_int2/2(DT_i)
  [e_Int2] -> Adaptive Law g#2_int2/4(e), Adaptive Law A#2_int2/6(e)
  [P_Int2] -> Adaptive Law g#2_int2/3(P), Adaptive Law A#2_int2/3(P)
  Module to compute Consensus Error #2_int2/1(ep) -> Memory4/1
  Memory4/1 -> Main Controller #2_int2/10(e_i), [e2_Int2]
  [x] -> Module to compute Consensus Error #2_int2/2(x)
  Dx0_hat_i/1 -> Differentiator1/1(x_d), Main Controller #2_int2/7(x0_hat_i), Adaptive Law A#2_int2/7(x0_hat_i), Module to compute Consensus Error #2_int2/3(x0)

== system CAMFC2_04_simple_DoubleIntegrator_02/Agent #2/Pendulum Plant #2/Plant ==
  U : Inport
  Clock : Clock
  Integrator : Integrator
  Integrator1 : Integrator
  Mux : Mux  Inputs=2
  Plant : MATLAB Function  TreatAsAtomicUnit=on
  Scope3 : Scope
  Y : Outport
  wires:
  Mux/1 -> Scope3/1, Y/1
  Clock/1 -> Plant/4(t)
  Plant/2(Dx2) -> Integrator1/1
  U/1 -> Plant/3(u)
  Integrator1/1 -> Mux/2, Plant/2(x2)
  Integrator/1 -> Mux/1, Plant/1(x1)
  Plant/1(Dx1) -> Integrator/1

== system CAMFC2_04_simple_DoubleIntegrator_02/Agent #3/Decenteralized Cooperaive Controller #3/Cooperative observer for formation variables #3 ==
  Agent_Num : Inport
  Integrator5 : Integrator  InitialCondition=zeros(N+1,n)
  Memory3 : Memory  InitialCondition=zeros(N+1,n)
  Observer T#3 : MATLAB Function  TreatAsAtomicUnit=on
  T_i : Outport
  tag scope: T3=global, epsilon3=global
  wires:
  Integrator5/1 -> T_i/1, [T3], Observer T#3/3(T_i)
  [T] -> Observer T#3/1(T)
  Memory3/1 -> [epsilon3]
  Observer T#3/1(DT_i) -> Integrator5/1
  [epsilon] -> Observer T#3/2(epsilon)
  Observer T#3/2(epsilon_i) -> Memory3/1
  Agent_Num/1 -> Observer T#3/4(Agent_Num)

== system CAMFC2_04_simple_DoubleIntegrator_02/Agent #3/Decenteralized Cooperaive Controller #3/Cooperative observer for leader states #3 ==
  Agent_Num : Inport
  Integrator6 : Integrator  InitialCondition=zeros(n0,1)
  Memory1 : Memory  InitialCondition=zeros(n0,1)
  Observer x0_hat#3 : MATLAB Function  TreatAsAtomicUnit=on
  x0_hat_i : Outport
  tag scope: x0_hat3=global, x0_tilde3=global
  wires:
  [x0_hat] -> Observer x0_hat#3/1(x0_hat)
  [x0_tilde] -> Observer x0_hat#3/2(x0_tilde)
  Integrator6/1 -> x0_hat_i/1, Observer x0_hat#3/3(x0_hat_i), [x0_hat3]
  Observer x0_hat#3/2(x0_tilde_i) -> Memory1/1
  Agent_Num/1 -> Observer x0_hat#3/5(Agent_Num)
  Memory1/1 -> [x0_tilde3]
  Observer x0_hat#3/1(Dx0_hat_i) -> Integrator6/1
  [x0] -> Observer x0_hat#3/4(x0)

== system CAMFC2_04_simple_DoubleIntegrator_02/Agent #3/Decenteralized Cooperaive Controller #3/Differentiator1 ==
  x_d : Inport
  Integrator : Integrator  InitialCondition=zeros(n0,1)
  Integrator1 : Integrator  InitialCondition=zeros(n0,1)
  Sliding differentiator : MATLAB Function  TreatAsAtomicUnit=on
  Sliding differentiator1 : MATLAB Function  TreatAsAtomicUnit=on
  Sum : Sum  Inputs=|-+
  Dx_d : Outport
  wires:
  Sliding differentiator/1(u) -> Integrator1/1, Dx_d/1
  Sliding differentiator1/1(Du1) -> Integrator/1
  Integrator/1 -> Sliding differentiator/1(u1)
  x_d/1 -> Sum/1
  Sum/1 -> Sliding differentiator/2(e), Sliding differentiator1/1(e)
  Integrator1/1 -> Sum/2

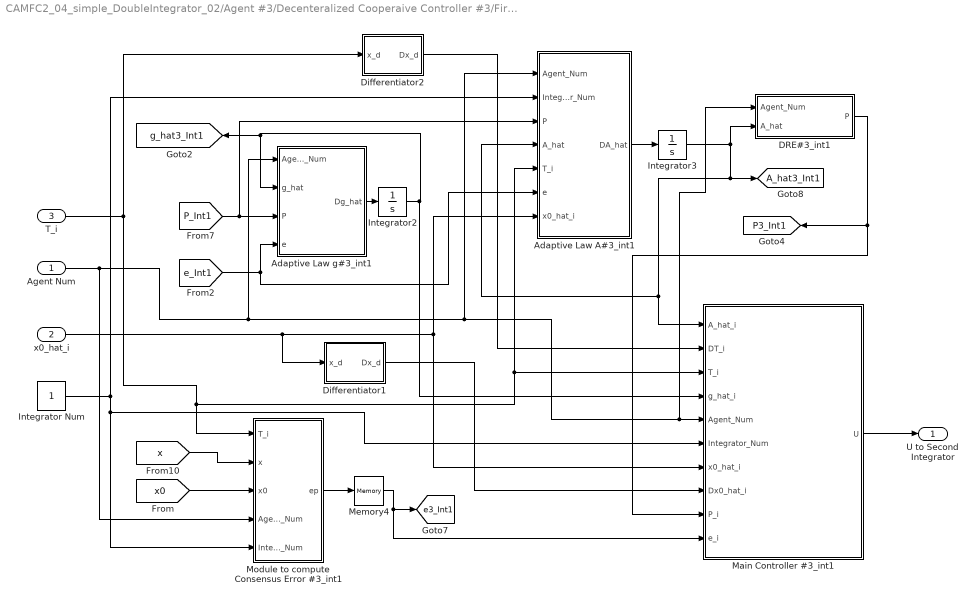
== system CAMFC2_04_simple_DoubleIntegrator_02/Agent #3/Decenteralized Cooperaive Controller #3/First Integrator #3 ==
  Agent Num : Inport
  x0_hat_i : Inport  Port=2
  T_i : Inport  Port=3
  Adaptive Law A#3_int1 : MATLAB Function  TreatAsAtomicUnit=on
  Adaptive Law g#3_int1 : MATLAB Function  TreatAsAtomicUnit=on
  DRE#3_int1 : Subsystem
  Differentiator1 : Subsystem
  Differentiator2 : Subsystem
  Integrator Num : Constant
  Integrator2 : Integrator  InitialCondition=zeros(n0,1)
  Integrator3 : Integrator  InitialCondition=zeros(n0)
  Main Controller #3_int1 : MATLAB Function  TreatAsAtomicUnit=on
  Memory4 : Memory  InitialCondition=zeros(n0,1)
  Module to compute Consensus Error #3_int1 : MATLAB Function  TreatAsAtomicUnit=on
  U to Second Integrator : Outport
  tag scope: A_hat3_Int1=global, P3_Int1=global, e3_Int1=global, g_hat3_Int1=global
  wires:
  DRE#3_int1/1(P) -> [P3_Int1], Main Controller #3_int1/9(P_i)
  Agent Num/1 -> Module to compute Consensus Error #3_int1/4(Agent_Num), Adaptive Law g#3_int1/1(Agent_Num), DRE#3_int1/1(Agent_Num), Main Controller #3_int1/5(Agent_Num), Adaptive Law A#3_int1/1(Agent_Num)
  Integrator2/1 -> Main Controller #3_int1/4(g_hat_i), Adaptive Law g#3_int1/2(g_hat), [g_hat3_Int1]
  Adaptive Law g#3_int1/1(Dg_hat) -> Integrator2/1
  Integrator3/1 -> DRE#3_int1/2(A_hat), Adaptive Law A#3_int1/4(A_hat), Main Controller #3_int1/1(A_hat_i), [A_hat3_Int1]
  Main Controller #3_int1/1(U) -> U to Second Integrator/1
  Adaptive Law A#3_int1/1(DA_hat) -> Integrator3/1
  Module to compute Consensus Error #3_int1/1(ep) -> Memory4/1
  [P_Int1] -> Adaptive Law A#3_int1/3(P), Adaptive Law g#3_int1/3(P)
  [e_Int1] -> Adaptive Law A#3_int1/6(e), Adaptive Law g#3_int1/4(e)
  [x0] -> Module to compute Consensus Error #3_int1/3(x0)
  Memory4/1 -> [e3_Int1], Main Controller #3_int1/10(e_i)
  [x] -> Module to compute Consensus Error #3_int1/2(x)
  Integrator Num/1 -> Main Controller #3_int1/6(Integrator_Num), Module to compute Consensus Error #3_int1/5(Integrator_Num), Adaptive Law A#3_int1/2(Integrator_Num)
  x0_hat_i/1 -> Differentiator1/1(x_d), Adaptive Law A#3_int1/7(x0_hat_i), Main Controller #3_int1/7(x0_hat_i)
  Differentiator1/1(Dx_d) -> Main Controller #3_int1/8(Dx0_hat_i)
  T_i/1 -> Adaptive Law A#3_int1/5(T_i), Main Controller #3_int1/3(T_i), Module to compute Consensus Error #3_int1/1(T_i), Differentiator2/1(x_d)
  Differentiator2/1(Dx_d) -> Main Controller #3_int1/2(DT_i)

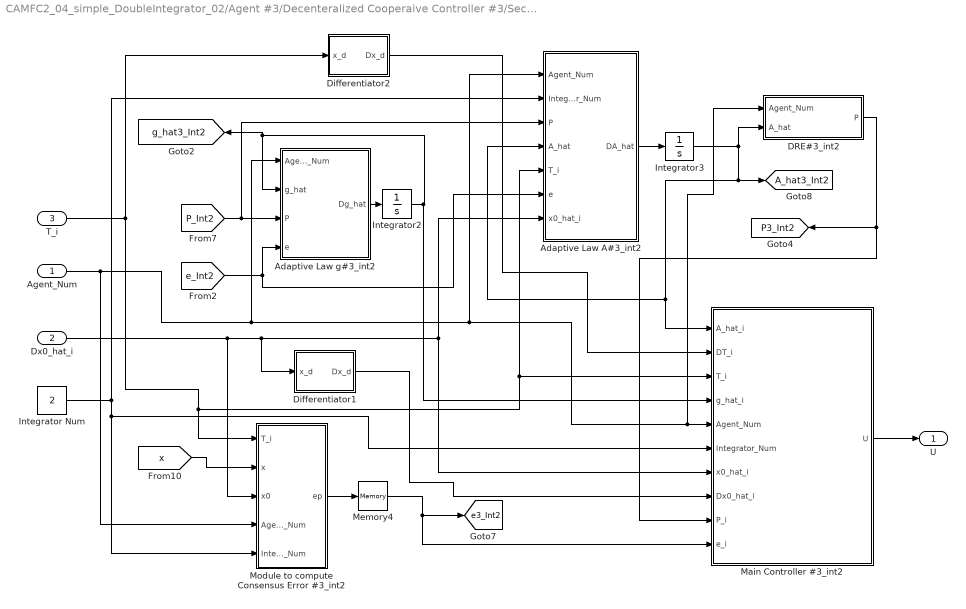
== system CAMFC2_04_simple_DoubleIntegrator_02/Agent #3/Decenteralized Cooperaive Controller #3/Second Integrator #3 ==
  Agent_Num : Inport
  Dx0_hat_i : Inport  Port=2
  T_i : Inport  Port=3
  Adaptive Law A#3_int2 : MATLAB Function  TreatAsAtomicUnit=on
  Adaptive Law g#3_int2 : MATLAB Function  TreatAsAtomicUnit=on
  DRE#3_int2 : Subsystem
  Differentiator1 : Subsystem
  Differentiator2 : Subsystem
  Integrator Num : Constant  Value=2
  Integrator2 : Integrator  InitialCondition=zeros(n0,1)
  Integrator3 : Integrator  InitialCondition=zeros(n0)
  Main Controller #3_int2 : MATLAB Function  TreatAsAtomicUnit=on
  Memory4 : Memory  InitialCondition=zeros(n0,1)
  Module to compute Consensus Error #3_int2 : MATLAB Function  TreatAsAtomicUnit=on
  U : Outport
  tag scope: A_hat3_Int2=global, P3_Int2=global, e3_Int2=global, g_hat3_Int2=global
  wires:
  [x] -> Module to compute Consensus Error #3_int2/2(x)
  Memory4/1 -> [e3_Int2], Main Controller #3_int2/10(e_i)
  Module to compute Consensus Error #3_int2/1(ep) -> Memory4/1
  [P_Int2] -> Adaptive Law A#3_int2/3(P), Adaptive Law g#3_int2/3(P)
  [e_Int2] -> Adaptive Law A#3_int2/6(e), Adaptive Law g#3_int2/4(e)
  Differentiator2/1(Dx_d) -> Main Controller #3_int2/2(DT_i)
  Adaptive Law A#3_int2/1(DA_hat) -> Integrator3/1
  Integrator3/1 -> DRE#3_int2/2(A_hat), Adaptive Law A#3_int2/4(A_hat), Main Controller #3_int2/1(A_hat_i), [A_hat3_Int2]
  Adaptive Law g#3_int2/1(Dg_hat) -> Integrator2/1
  Integrator2/1 -> Main Controller #3_int2/4(g_hat_i), Adaptive Law g#3_int2/2(g_hat), [g_hat3_Int2]
  Agent_Num/1 -> Module to compute Consensus Error #3_int2/4(Agent_Num), Adaptive Law g#3_int2/1(Agent_Num), DRE#3_int2/1(Agent_Num), Main Controller #3_int2/5(Agent_Num), Adaptive Law A#3_int2/1(Agent_Num)
  DRE#3_int2/1(P) -> [P3_Int2], Main Controller #3_int2/9(P_i)
  Differentiator1/1(Dx_d) -> Main Controller #3_int2/8(Dx0_hat_i)
  T_i/1 -> Differentiator2/1(x_d), Adaptive Law A#3_int2/5(T_i), Main Controller #3_int2/3(T_i), Module to compute Consensus Error #3_int2/1(T_i)
  Main Controller #3_int2/1(U) -> U/1
  Integrator Num/1 -> Main Controller #3_int2/6(Integrator_Num), Module to compute Consensus Error #3_int2/5(Integrator_Num), Adaptive Law A#3_int2/2(Integrator_Num)
  Dx0_hat_i/1 -> Adaptive Law A#3_int2/7(x0_hat_i), Main Controller #3_int2/7(x0_hat_i), Differentiator1/1(x_d), Module to compute Consensus Error #3_int2/3(x0)

== system CAMFC2_04_simple_DoubleIntegrator_02/Agent #3/Pendulum Plant #3/Plant ==
  U : Inport
  Clock : Clock
  Integrator : Integrator
  Integrator1 : Integrator
  Mux : Mux  Inputs=2
  Plant : MATLAB Function  TreatAsAtomicUnit=on
  Scope3 : Scope
  Y : Outport
  wires:
  Plant/1(Dx1) -> Integrator/1
  Integrator/1 -> Plant/1(x1), Mux/1
  Integrator1/1 -> Plant/2(x2), Mux/2
  U/1 -> Plant/3(u)
  Plant/2(Dx2) -> Integrator1/1
  Clock/1 -> Plant/4(t)
  Mux/1 -> Y/1, Scope3/1

== system CAMFC2_04_simple_DoubleIntegrator_02/Agent #4/Decenteralized Cooperaive Controller #4/Cooperative observer for formation variables #4 ==
  Agent_Num : Inport
  Integrator5 : Integrator  InitialCondition=zeros(N+1,n)
  Memory3 : Memory  InitialCondition=zeros(N+1,n)
  Observer T#4 : MATLAB Function  TreatAsAtomicUnit=on
  T_i : Outport
  tag scope: T4=global, epsilon4=global
  wires:
  Agent_Num/1 -> Observer T#4/4(Agent_Num)
  Observer T#4/2(epsilon_i) -> Memory3/1
  [epsilon] -> Observer T#4/2(epsilon)
  Memory3/1 -> [epsilon4]
  [T] -> Observer T#4/1(T)
  Integrator5/1 -> [T4], Observer T#4/3(T_i), T_i/1
  Observer T#4/1(DT_i) -> Integrator5/1

== system CAMFC2_04_simple_DoubleIntegrator_02/Agent #4/Decenteralized Cooperaive Controller #4/Cooperative observer for leader states #4 ==
  Agent_Num : Inport
  Integrator6 : Integrator  InitialCondition=zeros(n0,1)
  Memory1 : Memory  InitialCondition=zeros(n0,1)
  Observer x0_hat#4 : MATLAB Function  TreatAsAtomicUnit=on
  x0_hat_i : Outport
  tag scope: x0_hat4=global, x0_tilde4=global
  wires:
  [x0] -> Observer x0_hat#4/4(x0)
  Observer x0_hat#4/1(Dx0_hat_i) -> Integrator6/1
  Memory1/1 -> [x0_tilde4]
  Agent_Num/1 -> Observer x0_hat#4/5(Agent_Num)
  Observer x0_hat#4/2(x0_tilde_i) -> Memory1/1
  Integrator6/1 -> [x0_hat4], Observer x0_hat#4/3(x0_hat_i), x0_hat_i/1
  [x0_tilde] -> Observer x0_hat#4/2(x0_tilde)
  [x0_hat] -> Observer x0_hat#4/1(x0_hat)

== system CAMFC2_04_simple_DoubleIntegrator_02/Agent #4/Decenteralized Cooperaive Controller #4/Differentiator1 ==
  x_d : Inport
  Integrator : Integrator  InitialCondition=zeros(n0,1)
  Integrator1 : Integrator  InitialCondition=zeros(n0,1)
  Sliding differentiator : MATLAB Function  TreatAsAtomicUnit=on
  Sliding differentiator1 : MATLAB Function  TreatAsAtomicUnit=on
  Sum : Sum  Inputs=|-+
  Dx_d : Outport
  wires:
  Integrator1/1 -> Sum/2
  Sum/1 -> Sliding differentiator1/1(e), Sliding differentiator/2(e)
  x_d/1 -> Sum/1
  Integrator/1 -> Sliding differentiator/1(u1)
  Sliding differentiator1/1(Du1) -> Integrator/1
  Sliding differentiator/1(u) -> Dx_d/1, Integrator1/1
